simulink library "HighFrequencyNoiseEstimatorCoh"  (R2022b)
settings: Solver=VariableStepAuto  StartTime=0.0  StopTime=10.0  RelTol=1e-3
values from neighbouring files (symbols this model uses):
  NumAAChannels = NumHFRefChannels + 1    [HighFrequencyNoiseEstimatorCohMask.m]
  NumHFRefChannels = NumHFRefLPF + NumHFRefBPF    [HighFrequencyNoiseEstimatorCohMask.m]
undefined symbols (not defined in the file or in its folder): magnitude, Row
libraries: TuneVar x46, TOP x12, StateVar x10, FeaturePath x7, HandyTextFile x4, RfftLib x2, dspmathops x2, dspobslib x2, SpeedBoundsNoiseSlew x2, PooliirLib x2, TSP x1, dspsrcs4 x1
(part 2 of 2)

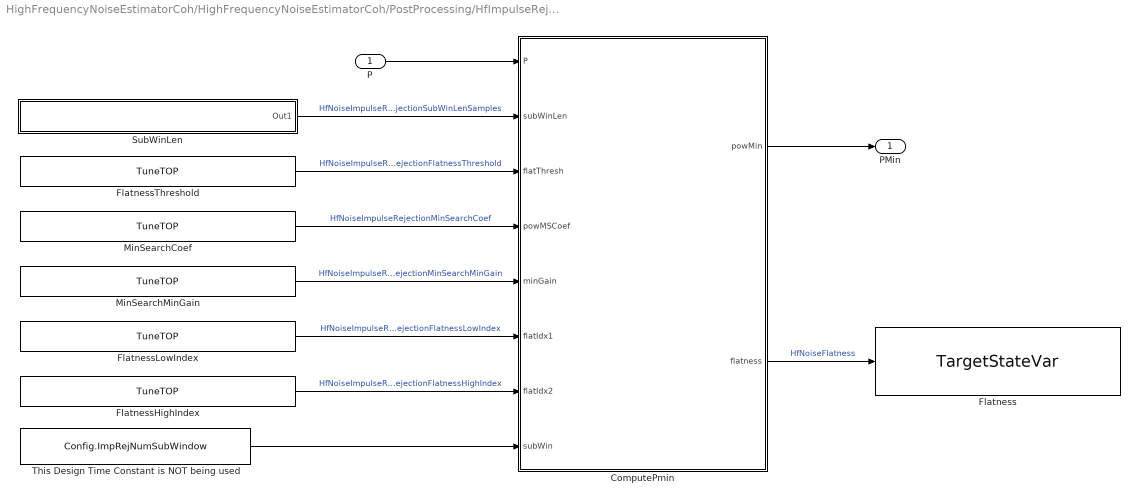
== system HighFrequencyNoiseEstimatorCoh/HighFrequencyNoiseEstimatorCoh/PostProcessing/HfImpulseRejection/MinSearch ==
  P : Inport
  ComputePmin : MATLAB Function  TreatAsAtomicUnit=on
  Flatness : StateVar/TargetStateVar  TriggerInit=[700 271 945 339]  TspName=Flatness  StateName=Flatness  UseSameName=on  IfdefMacro=[]
      settings: SourceProductName=Bose Talaria
  FlatnessHighIndex : TuneVar/TuneTOP  TriggerInit=[-155 320 120 350]  TopName=FlatnessHighIndex  TuneName=FlatnessHighIndex  DataType=single  TunabilityNumber=1  MinValue=[]  MaxValue=[]  BankNumber=0  PreOverlay=false  PostOverlay=false  UseSameName=on  MaskValue=Config.ImpRejFlatnessHighIndex
      settings: SourceProductName=Bose Talaria
  FlatnessLowIndex : TuneVar/TuneTOP  TriggerInit=[-155 265 120 295]  TopName=FlatnessLowIndex  TuneName=FlatnessLowIndex  DataType=single  TunabilityNumber=1  MinValue=[]  MaxValue=[]  BankNumber=0  PreOverlay=false  PostOverlay=false  UseSameName=on  MaskValue=Config.ImpRejFlatnessLowIndex
      settings: SourceProductName=Bose Talaria
  FlatnessThreshold : TuneVar/TuneTOP  TriggerInit=[-155 100 120 130]  TopName=FlatnessThresh  TuneName=FlatnessThresh  DataType=single  TunabilityNumber=1  MinValue=[]  MaxValue=[]  BankNumber=0  PreOverlay=false  PostOverlay=false  UseSameName=on  MaskValue=Config.ImpRejFlatnessThreshold
      settings: SourceProductName=Bose Talaria
  MinSearchCoef : TuneVar/TuneTOP  TriggerInit=[-155 155 120 185]  TopName=MinSearchCoef  TuneName=MinSearchCoef  DataType=single  TunabilityNumber=1  MinValue=[]  MaxValue=[]  BankNumber=0  PreOverlay=false  PostOverlay=false  UseSameName=on  MaskValue=Config.ImpRejMinSearchCoef
      settings: SourceProductName=Bose Talaria
  MinSearchMinGain : TuneVar/TuneTOP  TriggerInit=[-155 210 120 240]  TopName=MinSearchMinGain  TuneName=MinSearchMinGain  DataType=single  TunabilityNumber=1  MinValue=[]  MaxValue=[]  BankNumber=0  PreOverlay=false  PostOverlay=false  UseSameName=on  MaskValue=Config.ImpRejMinSearchMinGain
      settings: SourceProductName=Bose Talaria
  SubWinLen : Subsystem
  This Design Time Constant is NOT being used : Constant  Value=Config.ImpRejNumSubWindow  OutDataTypeStr=single
  PMin : Outport  VectorParamsAs1DForOutWhenUnconnected=off
  wires:
  This Design Time Constant is NOT being used/1 -> ComputePmin/8(subWin)
  ComputePmin/1(powMin) -> PMin/1
  P/1 -> ComputePmin/1(P)
  MinSearchCoef/1 -> ComputePmin/4(powMSCoef)  "HfNoiseImpulseRejectionMinSearchCoef"
  SubWinLen/1(Out1) -> ComputePmin/2(subWinLen)  "HfNoiseImpulseRejectionSubWinLenSamples"
  FlatnessLowIndex/1 -> ComputePmin/6(flatIdx1)  "HfNoiseImpulseRejectionFlatnessLowIndex"
  FlatnessThreshold/1 -> ComputePmin/3(flatThresh)  "HfNoiseImpulseRejectionFlatnessThreshold"
  FlatnessHighIndex/1 -> ComputePmin/7(flatIdx2)  "HfNoiseImpulseRejectionFlatnessHighIndex"
  MinSearchMinGain/1 -> ComputePmin/5(minGain)  "HfNoiseImpulseRejectionMinSearchMinGain"
  ComputePmin/2(flatness) -> Flatness/1  "HfNoiseFlatness"

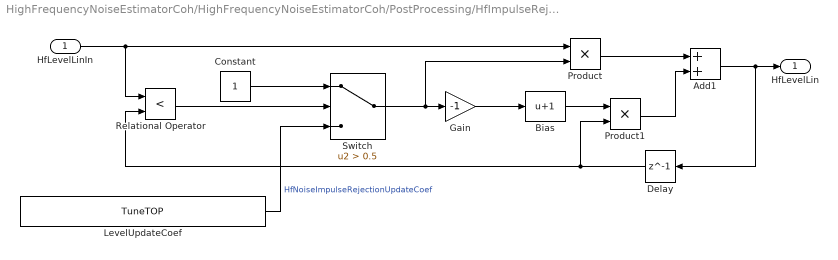
== system HighFrequencyNoiseEstimatorCoh/HighFrequencyNoiseEstimatorCoh/PostProcessing/HfImpulseRejection/SmoothingNoiseFloor ==
  HfLevelLinIn : Inport
  Add1 : Sum
  Bias : Bias  Bias=1  SaturateOnIntegerOverflow=off
  Constant : Constant  OutDataTypeStr=single
  Delay : Delay  DelayLength=1  InitialCondition=0.5
  Gain : Gain  Gain=-1
  LevelUpdateCoef : TuneVar/TuneTOP  TriggerInit=[20 280 265 310]  TopName=LevelUpdateCoef  TuneName=LevelUpdateCoef  DataType=single  TunabilityNumber=1  MinValue=[]  MaxValue=[]  BankNumber=0  PreOverlay=false  PostOverlay=false  UseSameName=on  MaskValue=Config.ImpRejLevelUpdateCoef
      settings: SourceProductName=Bose Talaria
  Product : Product  RndMeth=Zero
  Product1 : Product  RndMeth=Zero
  Relational Operator : RelationalOperator  Operator=<  OutDataTypeStr=boolean  InputSameDT=off
  Switch : Switch  Criteria=u2 > Threshold  Threshold=0.5  SaturateOnIntegerOverflow=off  InputSameDT=off
  HfLevelLin : Outport  VectorParamsAs1DForOutWhenUnconnected=off
  wires:
  Gain/1 -> Bias/1
  Delay/1 -> Relational Operator/2, Product1/2
  HfLevelLinIn/1 -> Relational Operator/1, Product/1
  Relational Operator/1 -> Switch/2
  Constant/1 -> Switch/1
  Switch/1 -> Gain/1, Product/2
  Bias/1 -> Product1/1
  Product/1 -> Add1/1
  Product1/1 -> Add1/2
  Add1/1 -> HfLevelLin/1, Delay/1
  LevelUpdateCoef/1 -> Switch/3  "HfNoiseImpulseRejectionUpdateCoef"

== system HighFrequencyNoiseEstimatorCoh/HighFrequencyNoiseEstimatorCoh/PostProcessing/HfSlew/attack ==
  TOP : TOP/TOP  TriggerInit=[200 107 420 153]  TopName=AttackDbPerSample  DataType=single  BankNumber=0  PreOverlay=false  PostOverlay=false  Role=Automatic
      settings: SourceProductName=Bose Talaria
  TranslateTrigger : TuneVar/TranslateTrigger  TriggerInit=[81 5 119 60]
      settings: SourceProductName=Bose Talaria
  Tune Variable : TuneVar/TuneVar  TuneName=AttackDbPerS  SpecifyMaxSize=off  VariableDim=1 (Row)  MaxSize=[1 1]  TunabilityNumber=1  MinValue=[]  MaxValue=[]  TriggerInit=[-300 105 -100 155]  MaskValue=Config.SlewAttackDbpersec
      settings: SourceProductName=Bose Talaria
  sec2sample : MATLAB Function  TreatAsAtomicUnit=on
  HfNoiseRefLatencySamples : Outport  VectorParamsAs1DForOutWhenUnconnected=off
  wires:
  TOP/1 -> HfNoiseRefLatencySamples/1  "AttackDbPerSample"
  sec2sample/1(y) -> TOP/1
  Tune Variable/1 -> sec2sample/1(u)  "AttackDbPerS"
  TranslateTrigger/1 -> sec2sample/Trigger

== system HighFrequencyNoiseEstimatorCoh/HighFrequencyNoiseEstimatorCoh/PostProcessing/HfSlew/decay ==
  TOP : TOP/TOP  TriggerInit=[200 110 395 150]  TopName=DecayDbPerSample  DataType=single  BankNumber=0  PreOverlay=false  PostOverlay=false  Role=Automatic
      settings: SourceProductName=Bose Talaria
  TranslateTrigger : TuneVar/TranslateTrigger  TriggerInit=[81 5 119 60]
      settings: SourceProductName=Bose Talaria
  Tune Variable : TuneVar/TuneVar  TuneName=DecayDbPerS  SpecifyMaxSize=off  VariableDim=1 (Row)  MaxSize=[1 1]  TunabilityNumber=1  MinValue=[]  MaxValue=[]  TriggerInit=[-300 110 -65 150]  MaskValue=Config.SlewDecayDbpersec
      settings: SourceProductName=Bose Talaria
  sec2sample : MATLAB Function  TreatAsAtomicUnit=on
  HfNoiseRefLatencySamples : Outport  VectorParamsAs1DForOutWhenUnconnected=off
  wires:
  TranslateTrigger/1 -> sec2sample/Trigger
  Tune Variable/1 -> sec2sample/1(u)  "DecayDbPerS"
  sec2sample/1(y) -> TOP/1
  TOP/1 -> HfNoiseRefLatencySamples/1  "DecayDbPerSample"

== system HighFrequencyNoiseEstimatorCoh/HighFrequencyNoiseEstimatorCoh/PostProcessing/HfImpulseRejection/MinSearch/SubWinLen ==
  Sec2Samples : MATLAB Function  TreatAsAtomicUnit=on
  TOP : TOP/TOP  TriggerInit=[5 25 270 75]  TopName=SubWinLenSamples  DataType=single  BankNumber=0  PreOverlay=false  PostOverlay=false  Role=Automatic
      settings: SourceProductName=Bose Talaria
  TranslateTrigger : TuneVar/TranslateTrigger  TriggerInit=[-129 -100 -91 -45]
      settings: SourceProductName=Bose Talaria
  Tune Variable : TuneVar/TuneVar  TuneName=SubWinTimeS  SpecifyMaxSize=off  VariableDim=1 (Row)  MaxSize=[1 1]  TunabilityNumber=1  MinValue=[]  MaxValue=[]  TriggerInit=[-520 25 -255 75]  MaskValue=Config.ImpRejSubWindowTimeSec
      settings: SourceProductName=Bose Talaria
  Out1 : Outport  VectorParamsAs1DForOutWhenUnconnected=off
  wires:
  TOP/1 -> Out1/1  "SubWinLenSamples"
  Tune Variable/1 -> Sec2Samples/1(time)  "SubWinTimeS"
  Sec2Samples/1(samples) -> TOP/1
  TranslateTrigger/1 -> Sec2Samples/Trigger

== matlab function HighFrequencyNoiseEstimatorCoh/PostProcessing/HfSlew/attack/sec2sample ==
  data: u input; y output; HFDecRate2 parameter
  events: trigger input FUNCTION_CALL_EVENT
function y = fcn(u, HFDecRate2)
% Convert rate from per sec to per sample

y = (u.Value/HFDecRate2);

== matlab function HighFrequencyNoiseEstimatorCoh/PostProcessing/HfSlew/decay/sec2sample ==
  data: u input; y output; HFDecRate2 parameter
  events: trigger input FUNCTION_CALL_EVENT
function y = fcn(u, HFDecRate2)
% Convert rate from per sec to per sample

y = -abs(u.Value/HFDecRate2);

== matlab function HighFrequencyNoiseEstimatorCoh/HfNoiseMusicSeparation /NoisePsdLevel/ExtractNoiseLevel ==
  data: PSD input; NoiseLevel output
  events: trigger input FUNCTION_CALL_EVENT
function NoiseLevel  = fcn(PSD)
% This sums the Power Spectral Density values across all
% frequency bands.
%#codegen

NoiseLevel = sum(PSD);

== matlab function HighFrequencyNoiseEstimatorCoh/RatioCalculation/APLFUP/LfNoiseUpdatePeriod/sec2samples ==
  data: samples output; time input; HFDecRate parameter
  events: trigger input FUNCTION_CALL_EVENT
function samples = fcn(time,HFDecRate)

% A trivial pass-through translation looks like this:
samples = ceil(time.Value*HFDecRate);

== matlab function HighFrequencyNoiseEstimatorCoh/RatioCalculation/RatioSmoother/RatioImpulseRejectionGamma0/Tau2Gamma ==
  data: gamma output; tau input; HFDecRate parameter
  events: trigger input FUNCTION_CALL_EVENT
function gamma  = Tau2Gamma(tau,HFDecRate)
% Approximate conversion from coefficient to time constant

wc = 1/(HFDecRate*tau.Value);
gamma = 1-(1-sin(wc))/cos(wc);

== matlab function HighFrequencyNoiseEstimatorCoh/RatioCalculation/RatioSmoother/RatioImpulseRejectionImpulseVarianceLpfCoef/Tau2Coef ==
  data: coef output; tau input; HFDecRate parameter
  events: trigger input FUNCTION_CALL_EVENT
function coef  = Tau2Coef(tau,HFDecRate)
% Convert from time constant to 1st order coefficient
%#codegen

wc = 1/(HFDecRate*tau.Value);
coef = (1-sin(wc))/cos(wc);

== matlab function HighFrequencyNoiseEstimatorCoh/RatioCalculation/RatioSmoother/RatioSmoother ==
  data: UpdateFlag input; PreRatioLinear input; RatioCoef input size=1 =ratioCoef; RatioFiltCoef input =ratioFiltCoef; NoiseScale input =noiseScale; ImpulseScale input =impulseScale; GammaCorr input =gammaCorr; PreRatioMin input; RatioLinear output; ImpRejFiltOutInit input
function RatioLinear = RatioSmoother(UpdateFlag, PreRatioLinear, ...
	RatioCoef, ...
	RatioFiltCoef, ...
	NoiseScale, ...
	ImpulseScale, ...
	GammaCorr, ...
	PreRatioMin, ...
	ImpRejFiltOutInit)

persistent PreRatioLinLP ImpFiltState ImpRejFiltOut;
if isempty(PreRatioLinLP); PreRatioLinLP = single(0); end
if isempty(ImpFiltState); ImpFiltState = single([0 0]);	end
if isempty(ImpRejFiltOut); ImpRejFiltOut = single(ImpRejFiltOutInit); end

% Energy Conversion
PreRatioLinLP = PreRatioLinLP*RatioCoef ...
    + abs(PreRatioLinear)*(1-RatioCoef);

% Instantaneous Noise Estimate
RatioInstant = abs(PreRatioLinLP);

% Impulse Estimate
% Double application of 1st order LPF (A Dublin hack)
ImpFiltState(1) = ImpFiltState(1)*RatioFiltCoef ...
    + RatioInstant*(1-RatioFiltCoef);
ImpFiltState(2) = ImpFiltState(2)*RatioFiltCoef ...
    + ImpFiltState(1)*(1-RatioFiltCoef);

% Variances
noiseVar = NoiseScale * ImpFiltState(2)^2;
impulseVar = ImpulseScale ...
    * (min(0,RatioInstant-ImpFiltState(2)))^2;
totalVar = noiseVar + max(0,impulseVar);

% Gamma correction
impRejFiltCoef = (1 - GammaCorr*noiseVar/(totalVar+eps));

% Impulse Reject Filter
% If the new value is larger than the current value, use the new value for
% update.  Otherwise, if the new value is smaller, then update only if the
% update flag is also raised.
if (RatioInstant >= ImpRejFiltOut) || ((RatioInstant < ImpRejFiltOut)&& UpdateFlag)
    ImpRejFiltOut = impRejFiltCoef*ImpRejFiltOut+RatioInstant*(1-impRejFiltCoef);
end

% dBSPL Conversion and microphone energy check
RatioLinear = max(ImpRejFiltOut+eps, PreRatioMin);
return

== matlab function HighFrequencyNoiseEstimatorCoh/RatioCalculation/EnergyLpfCoef/Tau2Coef ==
  data: coef output; tau input; HFDecRate parameter
  events: trigger input FUNCTION_CALL_EVENT
function coef  = Tau2Coef(tau,HFDecRate)
% Convert from time constant to 1st order coefficient
%#codegen

wc = 1/(HFDecRate*tau.Value);
coef = (1-sin(wc))/cos(wc);

== matlab function HighFrequencyNoiseEstimatorCoh/PostProcessing/HfImpulseRejection/MinSearch/SubWinLen/Sec2Samples ==
  data: samples output; time input; HFDecRate2 parameter
  events: trigger input FUNCTION_CALL_EVENT
function samples  = Sec2Samples(time,HFDecRate2)
% Convert period in sec to samples
%#codegen

samples = ceil(HFDecRate2*time.Value);

== matlab function HighFrequencyNoiseEstimatorCoh/HfNoiseMusicSeparation /GaussianElimination/If Action Subsystem/CoherenceModifier ==
  data: u input; u output
function u = CoherenceModifier(u)
%#eml
% For coherence that is higher than threshold (meaning noise is low), we will enhance it to avoid
% overestimation at low noise level
N = length(u);
threshold = 0.88;
%y = u;
for i = 1:N
    if u(i) > threshold 
        u(i) = sqrt((u(i)-threshold)*(1-threshold)) + threshold;
    end
end

== matlab function HighFrequencyNoiseEstimatorCoh/HfNoiseMusicSeparation /RefPowerMin/undB ==
  data: TOP output; Tune input
  events: trigger input FUNCTION_CALL_EVENT
function TOP  = fcn(Tune)
%#codegen

TOP = undb20(Tune.Value);

== matlab function HighFrequencyNoiseEstimatorCoh/HfNoiseMusicSeparation /MicPsdLevel/ExtractMicLevel ==
  data: CSD input; MicLevel output
function MicLevel = fcn(CSD)
% This function generates a microphone level by 
% (1) Extracting Gyy from the cross-spectral density matrix
%     It is the last entry (last column, last row) of the matrix.
% (2) Sum Gyy over all frequency bands

Gyy = CSD(:,end,end);
MicLevel = sum(Gyy);

== matlab function HighFrequencyNoiseEstimatorCoh/HfNoiseMusicSeparation /GaussianElimination/If Action Subsystem/GaussianElimination ==
  data: c output; Gyy output; GXY input
function [c,Gyy] = GaussianElimination(GXY)
%#eml

% global GXY;

u = GXY;
M = size(u,1);  % Number of frequency bins
N = size(u,2);  % Size of coherence matrix

% Vectors of Noise
c = single(zeros(M,1));
Gyy = real(u(:,N,N));

for i = 1:M
    % Loop over each frequency bin
    S_data = squeeze(u(i,:,:));
    S_mod = GaussianElim(S_data);
    Snn_Gauss = S_mod(N,N);
    %Gnn(i) = real(Snn_Gauss);
     if S_data(N,N) > eps
        c(i) = 1-real(Snn_Gauss)/real(S_data(N,N));
     else
        c(i) = 1;
     end
end
end

function b = GaussianElim(a)
% This function performs Gaussian elimination 
% on a cross-correlation matrix, a. 
temp = a;
m = size(a,1);
for j =1:m-1
   for i = j+1:m
       if ((j>1) && abs(a(j,j)/temp(j,j)) > 0.001) || ((j==1) && abs(a(j,j))>eps)
           % starting from 2nd row, if the conditioned psd is close to
           % zero, we should skip using this row for the next elimination
           % operation; similarly if the first input (G11) is zero, we
           % should skip using the first row
           
           mult = a(i,j)/a(j,j);
           a(i,:) = a(i,:)-a(j,:)*mult;
       end
   end
end
b = a;
end

== matlab function HighFrequencyNoiseEstimatorCoh/RatioCalculation/RatioSlew/decay/sec2sample ==
  data: u input; y output; HFDecRate parameter
  events: trigger input FUNCTION_CALL_EVENT
function y = RateConversion(u, HFDecRate)
% Convert rate from per sec to per sample

y = -abs(u.Value/HFDecRate);

== matlab function HighFrequencyNoiseEstimatorCoh/RatioCalculation/APLFUP/FlagHoldTime/sec2samples ==
  data: samples output; time input; HFDecRate parameter
  events: trigger input FUNCTION_CALL_EVENT
function samples  = fcn(time,HFDecRate)
%#codegen

samples = ceil(time.Value*HFDecRate);

== matlab function HighFrequencyNoiseEstimatorCoh/HfNoiseMusicSeparation /FormCoherenceMatrixGXY ==
  data: GnnUpdate output; StftIn input; HFWELCHSIZE input; GXYOut output
function [GnnUpdate,GXYOut] = FormGXY(StftIn,HFWELCHSIZE)

K = HFWELCHSIZE;               % K: size of Welch window
L = ceil(size(StftIn,1)/2);    % L: number frequency bins
M = size(StftIn,2);            % M: mic + number of ref channels

persistent GXY;
persistent frame_counter;

% Initialize states
if isempty(GXY) 
    GXY=complex(single(zeros(L,M,M))); 
end
if isempty(frame_counter) 
    frame_counter=int16(0); 
end

% Modulo K Counter
if frame_counter < K
    % frame counter increment
    frame_counter = frame_counter + int16(1);
else        
    % reset frame counter
    frame_counter = int16(1);
end

%#codegen
if frame_counter < K
    % Reset at the first frame
    if frame_counter == 1
        GXY = complex(single(zeros(L,M,M)));
    end
    % Accumulate
    for i = 1:M
        for j = i:M
            % Loop over the lower triangular matrix (including the diagonal)
            EXY = (conj((2*StftIn(1:2:end,i)))) .* (2*StftIn(1:2:end,j)); 
            GXY(:,i,j) = GXY(:,i,j)+ EXY/K;
        end
    end
    GnnUpdate = false; 
else
    % Last Frame
    for i = 1:M
        for j = i:M
            % Loop over the lower triangular matrix (including the diagonal)
            EXY = (conj((2*StftIn(1:2:end,i)))) .* (2*StftIn(1:2:end,j));
            GXY(:,i,j) = GXY(:,i,j)+ EXY/K;
        end
        for j = 1:i-1
            % Construct full matrix when Welch window size is met
            GXY(:,i,j) = conj(GXY(:,j,i));
        end
    end
    GnnUpdate = true; 
end
GXYOut = GXY;

== matlab function HighFrequencyNoiseEstimatorCoh/HfNoiseMusicSeparation /GnnInitNoiseFloor ==
  data: RefPowerMin input; Gnn data_store_memory
function fcn(RefPowerMin)
% Initialize noise floor in Gnn based on ref_pow_min TOP 

persistent init_noise_floor;  % Flag
global Gnn;

% Initialize the flag
if isempty(init_noise_floor) 
    init_noise_floor = false;
end

% Initialize Gnn
if(~init_noise_floor)
   Gnn(:) = RefPowerMin;
   init_noise_floor = true;
end

== matlab function HighFrequencyNoiseEstimatorCoh/PostProcessing/HfImpulseRejection/MinSearch/ComputePmin ==
  data: P input; powMin output single; subWinLen input; flatThresh input; powMSCoef input; minGain input; flatIdx1 input; flatIdx2 input; subWin input; flatness output
function [powMin, flatness] = MinSearch(P, ...
	subWinLen, ...
	flatThresh, ...
	powMSCoef, ...
	minGain, ...
	flatIdx1, ...
	flatIdx2, ...
	subWin)

numFreqBins = size(P,1);

% Because of restrictions on vsriable-size arrays, this number is currently
% hard-coded. It is intended to be subWin.
numSubWin = 3;
% The minimum value of 1e-8, currently hard-coded, should also be variable
% or globally defined.

persistent IRMinCount IRSubMin IRPowMS;
if isempty(IRMinCount);	IRMinCount	= single(-1); end
if isempty(IRSubMin);	IRSubMin	= single(ones(numSubWin, numFreqBins))*1e-8;	end
if isempty(IRPowMS);	IRPowMS		= single(ones(1, numFreqBins))*1e-8;	end

% The following is a low-storage method for calculating a running minimum
% over a sliding window
IRMinCount = mod(IRMinCount + 1, numSubWin*subWinLen);
currentSubWin = floor(IRMinCount / subWinLen) + 1;

if mod(IRMinCount, subWinLen) == 0
	IRSubMin(currentSubWin, :) = 1;
end

IRSubMin(currentSubWin, :) = min(IRSubMin(currentSubWin, :), P.');
IRGlobalMin = min(IRSubMin); 

% Flatness Calculations
% Geometric mean over arithmatic mean
flatness = 10^(mean(log10(IRGlobalMin(flatIdx1:flatIdx2)))) / ...
	(mean(IRGlobalMin(flatIdx1:flatIdx2))+eps);

if flatness >= flatThresh
	% accept new value
    IRPowMS = powMSCoef*IRPowMS + (1-powMSCoef)*IRGlobalMin; 
else 
	% else, take the smaller of the current sample and the storage
    IRPowMS = min(IRPowMS, IRGlobalMin); 
end

powMin = single(IRPowMS.'*minGain);

end

== matlab function HighFrequencyNoiseEstimatorCoh/ReferenceLatency/RefLatency/ms2samples ==
  data: DelayTimeMS input; MaxLatencySamples input; Samples output; HFDecRate parameter
  events: trigger input FUNCTION_CALL_EVENT
function Samples = fcn(DelayTimeMS, MaxLatencySamples, HFDecRate)
% Convert from time constant to samples

Samples = floor(DelayTimeMS.Value*HFDecRate/1000);
% Use floor to minimize the risk of going noncausal 

if Samples > MaxLatencySamples
    TranslateError('Delay amount cannot be greater than specified max delay');
end

== matlab function HighFrequencyNoiseEstimatorCoh/RatioCalculation/RatioSlew/attack/sec2sample ==
  data: u input; y output; HFDecRate parameter
  events: trigger input FUNCTION_CALL_EVENT
function y = fcn(u, HFDecRate)
% Convert rate from per sec to per sample

y = abs(u.Value/HFDecRate);

== matlab function HighFrequencyNoiseEstimatorCoh/RatioCalculation/APLFUP/APLFUP ==
  data: LF input; HF input; LFUPFlag output; speed input; noiseUpThresh input; HoldTime1 input; HoldTime2 input; SpeedThresh input; LFUPThresh input; HFUPThresh input
function LFUPFlag = fcn(LF, HF, speed, ...
 noiseUpThresh, ...
 HoldTime1, ...
 HoldTime2, ...
 SpeedThresh, ...
 LFUPThresh, ...
 HFUPThresh)
% This function is to check if the low freq noise goes up when the high
% freq noise is going up. Only when both noise go up, the flag is set to
% enable the ratio change and tuning adjustment
%#eml
persistent prev counter counter2 LFUP;

if isempty(prev);		prev = single(0);		end
if isempty(counter);	counter = single(0);	end
if isempty(counter2);	counter2 = single(0);	end
if isempty(LFUP);		LFUP = single(0);		end

if ((LF >= prev + noiseUpThresh) && (speed >= SpeedThresh))
	LFUP = single(1);
	counter = single(0); 
    % If low freq noise goes up by more than noiseUpThresh dB and the speed
    % is above the SpeedThresh, set the flag ON and reset the counter, this
    % is usually the case when the windows roll down
elseif (LFUP == 1) && (counter < HoldTime1)
	counter = counter + 1;
    % elseif the flag is ON and the hold period has not expired, update the
    % counter for hold time1
else
	LFUP = single(0);
	counter = single(0);
    % else, reset the flag and the counter
end

if (LF > LFUPThresh) && (speed >= SpeedThresh) || (HF > HFUPThresh) 
	LFUP = single(1);
	counter = HoldTime1 - 2;
    % In another case, if the low freq noise level is above LFUPThresh and
    % the high freq noise is above HFUPThresh and the speed is above
    % SpeedThresh, set the flag ON. This usually happens when the window is
    % already down and vehicle starts to speed up
end

% to prevent too small variations in low freq noise, we only update the low
% freq noise reading every HoldTime2 seconds.
if counter2 == HoldTime2 - 1
	prev = LF;
	counter2 = single(0);
else
	counter2 = counter2 + 1;
end

LFUPFlag = LFUP;
